simulink model "VehicleFollowing"  (R2020b)
settings: Solver=FixedStepAuto  StartTime=0.0  StopTime=23  FixedStep=Ts/2  RelTol=1e-3
PreLoadFcn:
  | VehicleFollowingInit;
values from neighbouring files (symbols this model uses):
  a_max = 2    [VehicleFollowingInit.m]
  a_min = -3    [VehicleFollowingInit.m]
  dimensionsEgo = [4; 2]    [VehicleFollowingInit.m]
  dimensionsLead = [6; 2]    [VehicleFollowingInit.m]
  dLead = 0    [VehicleFollowingInit.m]
  laneWidth = 3.7    [VehicleFollowingInit.m]
  lookAheadDistance = 6    [VehicleFollowingInit.m]
  roadTrajectory = [s_min  0        0 ... (first row only)    [VehicleFollowingInit.m]
  sLead_0 = 60    [VehicleFollowingInit.m]
  Ts = 0.01    [VehicleFollowingInit.m]    (also in prepare_simulation.m)
  v_max = 30    [VehicleFollowingInit.m]
  v_min = 0    [VehicleFollowingInit.m]
  vEgo_0 = 15    [VehicleFollowingInit.m]
  vLead_0 = 10    [VehicleFollowingInit.m]
  vLead_ref = vLead_0    (= 10)    [VehicleFollowingInit.m]
  wheelBaseEgo = 3    [VehicleFollowingInit.m]
  wheelBaseLead = 4    [VehicleFollowingInit.m]
  xEgo_0 = positionEgo_0(1)    [VehicleFollowingInit.m]
  xLead_0 = positionLead_0(1)    [VehicleFollowingInit.m]
  yEgo_0 = positionEgo_0(2)    [VehicleFollowingInit.m]
  yLead_0 = positionLead_0(2)    [VehicleFollowingInit.m]
undefined symbols (not defined in the file or in its folder): yawEgo_0, yawLead_0
libraries: pid_lib x2, sim3dautolib x2, vrlib x2, simulink x2, robotmobilelib x1, robotalgslib x1, drivingvehiclecontroller x1, sim3dlib x1, mpcadaslib x1
settings Model: Creator=Mustafa  LastModifiedBy=manuel
settings SFSimCC: CustomCodeUndefinedFunction=UseInterfaceOnly

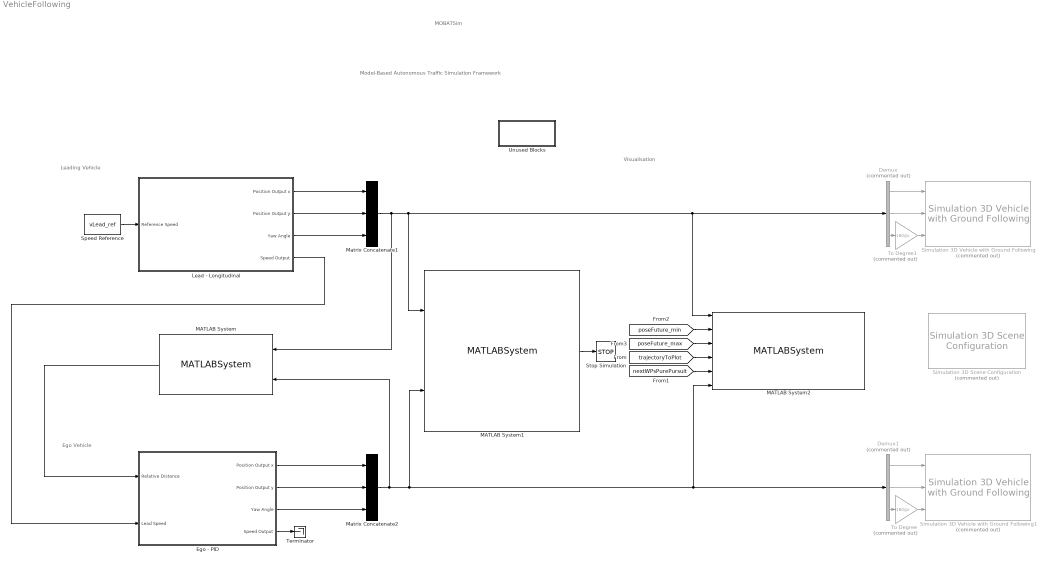
== system VehicleFollowing ==
  note: Visualisation
  note: Leading Vehicle
  note: Model-Based Autonomous Traffic Simulation Framework
  note: MOBATSim
  note: Ego Vehicle
  Demux : Demux  Commented=on  Outputs=3
  Demux1 : Demux  Commented=on  Outputs=3
  Ego - PID : Subsystem  mask{Speed=vEgo_0}
      mask prompts: Speed "Initial Speed"
      mask TypeOptions Speed: Initial Speed/Value
  Lead - Longitudinal : Subsystem  mask{s_0=sLead_0, d=dLead, Speed=vLead_0}
      mask prompts: s_0 "Initial s (Frenet)"; d "d (Frenet)"; Speed "Initial Speed"
      mask TypeOptions s_0: Initial Frenet s-coordinate/Value
      mask TypeOptions d: Frenet d-coordinate/Value
      mask TypeOptions Speed: Initial Speed/Value
  MATLAB System : MATLABSystem  System=RelativeFrenetDistance  LaneWidth=laneWidth  RoadTrajectory=roadTrajectory  SimulateUsing=Interpreted execution
      mask Type: RelativeFrenetDistance
      mask Display:
      | disp('RelativeFrenetDistance');
      | port_label('input',1,'poseLead');
      | port_label('input',2,'poseEgo');
      | port_label('output',1,'deltaS');
  MATLAB System1 : MATLABSystem  System=CollisionDetection  dimensionsEgo=dimensionsEgo  wheelBaseEgo=wheelBaseEgo  radiusEgo=radiusEgo  dimensionsLead=dimensionsLead  wheelBaseLead=wheelBaseLead  radiusLead=radiusLead  SimulateUsing=Interpreted execution
      mask Type: CollisionDetection
      mask Display:
      | disp('CollisionDetection');
      | port_label('input',1,'poseLead');
      | port_label('input',2,'poseEgo');
      | port_label('output',1,'collisionDetected');
  MATLAB System2 : MATLABSystem  System=PlotDrivingScenario  dimensionsLead=dimensionsLead  wheelBaseLead=wheelBaseLead  dimensionsEgo=dimensionsEgo  wheelBaseEgo=wheelBaseEgo  LaneWidth=laneWidth  RoadTrajectory=roadTrajectory  spaceDiscretisationMatrix=spaceDiscretisationMatrix  SimulateUsing=Interpreted execution
      mask Type: PlotDrivingScenario
      mask Display:
      | disp('PlotDrivingScenario');
      | port_label('input',1,'poseLead');
      | port_label('input',2,'poseLeadFuture_min');
      | port_label('input',3,'poseLeadFuture_max');
      | port_label('input',4,'egoTrajectory');
      | port_label('input',5,'nextWPsPurePursuit');
      | port_label('input',6,'poseEgo');
  Matrix Concatenate1 : Concatenate  NumInputs=3  ConcatenateDimension=2
  Matrix Concatenate2 : Concatenate  NumInputs=3  ConcatenateDimension=2
  Simulation 3D Scene Configuration : sim3dlib/Simulation 3D Scene Configuration  Priority=0  Commented=on  ProjectFormat=Default Scenes  SceneDesc=Straight road  ProjectName=VehicleSimulation.exe  ScenePath=/Game/Maps/HwStrght  vehTagList={'Scene Origin';'SimulinkVehicle1';'SimulinkVehicle2'}  vehTag=SimulinkVehicle2  OpVisEn=off  Ts=0.1  EnableWindow=on  sensorTag=MainCamera1  sensorId=1  sensorName=MainCamera1  mountLoc=Origin  offsetFlag=off  tmountOffset=[0, 0, 0]  rmountOffset=[0, 0, 0]  HorizontalResolution=1280  VerticalResolution=720  HorizontalFOV=60  mountPoint=[0 0 0]  mountOrientation=[0 0 0]  aMode=3  ID=1
      settings: SourceProductBaseCode=DR,UV,VE
  Simulation 3D Vehicle with Ground Following : sim3dautolib/Simulation 3D Vehicle with Ground Following  Priority=-1  Commented=on  PassVehMesh=Small pickup truck  VehColor=Orange  InitialPos=[xLead_0, yLead_0, yawLead_0]  InitialRot=[0, 0, 0]  ActorName=SimulinkVehicle1  SampleTime=0.1  ActorType=SimulinkVehicle  ID=1  aMode=3  ActorTag=SimulinkVehicle1  CoordinateScheme=ISO  TransformOutportEnabled=off
      settings: SourceProductBaseCode=DR,UV,VE
  Simulation 3D Vehicle with Ground Following1 : sim3dautolib/Simulation 3D Vehicle with Ground Following  Priority=-1  Commented=on  PassVehMesh=Muscle car  VehColor=Red  InitialPos=[xEgo_0, yEgo_0, yawEgo_0]  InitialRot=[0, 0, 0]  ActorName=SimulinkVehicle2  SampleTime=0.1  ActorType=SimulinkVehicle  ID=2  aMode=3  ActorTag=SimulinkVehicle2  CoordinateScheme=ISO  TransformOutportEnabled=off
      settings: SourceProductBaseCode=DR,UV,VE
  Speed Reference : Constant  Value=vLead_ref
  Stop Simulation : Stop
  Terminator : Terminator
  To Degree : Gain  Commented=on  Gain=180/pi
  To Degree1 : Gain  Commented=on  Gain=180/pi
  Unused Blocks : Subsystem
  wires:
  Speed Reference/1 -> Lead - Longitudinal/1(Reference Speed)
  Ego - PID/1(Position Output x) -> Matrix Concatenate2/1
  MATLAB System/1 -> Ego - PID/1(Relative Distance)
  Ego - PID/4(Speed Output) -> Terminator/1
  Ego - PID/2(Position Output y) -> Matrix Concatenate2/2
  Ego - PID/3(Yaw Angle) -> Matrix Concatenate2/3
  Matrix Concatenate1/1 -> Demux/1, MATLAB System2/1, MATLAB System1/1, MATLAB System/1
  Demux/1 -> Simulation 3D Vehicle with Ground Following/1
  Demux/2 -> Simulation 3D Vehicle with Ground Following/2
  Matrix Concatenate2/1 -> MATLAB System1/2, MATLAB System2/6, Demux1/1, MATLAB System/2
  Demux1/1 -> Simulation 3D Vehicle with Ground Following1/1
  Demux1/2 -> Simulation 3D Vehicle with Ground Following1/2
  Demux1/3 -> To Degree/1
  To Degree/1 -> Simulation 3D Vehicle with Ground Following1/3
  MATLAB System1/1 -> Stop Simulation/1
  Demux/3 -> To Degree1/1
  To Degree1/1 -> Simulation 3D Vehicle with Ground Following/3
  Lead - Longitudinal/1(Position Output x) -> Matrix Concatenate1/1
  Lead - Longitudinal/4(Speed Output) -> Ego - PID/2(Lead Speed)
  Lead - Longitudinal/3(Yaw Angle) -> Matrix Concatenate1/3
  Lead - Longitudinal/2(Position Output y) -> Matrix Concatenate1/2
  [nextWPsPurePursuit] -> MATLAB System2/5
  [trajectoryToPlot] -> MATLAB System2/4
  [poseFuture_min] -> MATLAB System2/2
  [poseFuture_max] -> MATLAB System2/3

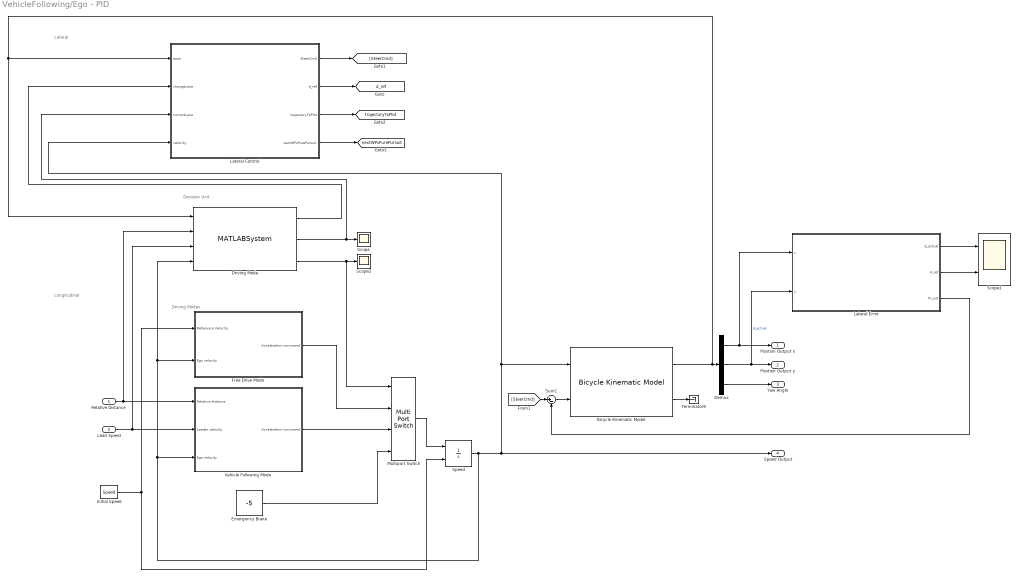
== system VehicleFollowing/Ego - PID ==
  note: Decision Unit
  note: Driving Modes
  note: Longitudinal
  note: Lateral
  Relative Distance : Inport
  Lead Speed : Inport  Port=2
  Bicycle Kinematic Model : robotmobilelib/Bicycle Kinematic Model  VehicleInputs=Vehicle Speed & Steering Angle  WheelBase=wheelBaseEgo  VehicleSpeedRange=[v_min v_max]  MaxSteeringAngle=steerAngle_max  InitialState=[xEgo_0; yEgo_0; yawEgo_0]  SimulateUsing=Interpreted execution
      settings: SourceProductBaseCode=RO
  Demux : Demux  Outputs=3
  Driving Mode : MATLABSystem  System=Decision  LaneWidth=laneWidth  RoadTrajectory=roadTrajectory  SimulateUsing=Interpreted execution
      mask Type: Decision
      mask Display:
      | disp('Decision');
      | port_label('input',1,'poseEgo');
      | port_label('input',2,'deltaS');
      | port_label('input',3,'vLead');
      | port_label('input',4,'vEgo');
      | port_label('output',1,'changeLaneCmd');
      | port_label('output',2,'currentLane');
      | port_label('output',3,'drivingMode');
  Emergency Brake : Constant  Value=-5
  Free Drive Mode : Subsystem
  Initial Speed : Constant  Value=Speed
  Lateral Control : Subsystem  Variant=on  VariantControlMode=label  LabelModeActiveChoice=STANLEY  mask{modeLateral=STANLEY}
      mask prompts: modeLateral "Lateral Mode:"
      mask TypeOptions modeLateral: PURE_PURSUIT | STANLEY
      mask Callback modeLateral: set_param(gcb,'OverrideUsingVariant',get_param(gcb,'modeLateral'))
  Lateral Error : Subsystem
  Multiport Switch : MultiPortSwitch
  Scope : Scope
  Scope1 : Scope  NumInputPorts=2
  Scope2 : Scope
  Speed : Integrator  InitialConditionSource=external  LimitOutput=on  UpperSaturationLimit=v_max  LowerSaturationLimit=v_min
  Sum1 : Sum  Inputs=|+-
  Terminator9 : Terminator
  Vehicle Following Mode : Subsystem
  Position Output x : Outport  VectorParamsAs1DForOutWhenUnconnected=off
  Position Output y : Outport  Port=2  VectorParamsAs1DForOutWhenUnconnected=off
  Yaw Angle : Outport  Port=3  VectorParamsAs1DForOutWhenUnconnected=off
  Speed Output : Outport  Port=4  VectorParamsAs1DForOutWhenUnconnected=off
  tag scope: d_ref=global, nextWPsPurePursuit=global, trajectoryToPlot=global
  wires:
  Initial Speed/1 -> Free Drive Mode/1(Reference Velocity), Speed/2
  Relative Distance/1 -> Driving Mode/2, Vehicle Following Mode/1(Relative distance)
  Lead Speed/1 -> Driving Mode/3, Vehicle Following Mode/2(Leader velocity)
  Vehicle Following Mode/1(Acceleration command) -> Multiport Switch/3
  Multiport Switch/1 -> Speed/1
  Free Drive Mode/1(Acceleration command) -> Multiport Switch/2
  Emergency Brake/1 -> Multiport Switch/4
  Driving Mode/3 -> Scope2/1, Multiport Switch/1
  Demux/3 -> Yaw Angle/1
  Bicycle Kinematic Model/2 -> Terminator9/1
  Demux/2 -> Position Output y/1, Lateral Error/2(y)  "d_actual"
  Driving Mode/2 -> Lateral Control/3(currentLane), Scope/1
  Lateral Control/1(SteerCmd) -> [SteerCmd]
  Lateral Control/2(d_ref) -> [d_ref]
  Driving Mode/1 -> Lateral Control/2(changeLane)
  Speed/1 -> Speed Output/1, Lateral Control/4(velocity), Bicycle Kinematic Model/1, Vehicle Following Mode/3(Ego velocity), Free Drive Mode/2(Ego velocity), Driving Mode/4
  Bicycle Kinematic Model/1 -> Driving Mode/1, Lateral Control/1(pose), Demux/1
  Lateral Control/3(trajectoryToPlot) -> [trajectoryToPlot]
  Lateral Control/4(nextWPsPurePursuit) -> [nextWPsPurePursuit]
  Sum1/1 -> Bicycle Kinematic Model/2
  [SteerCmd] -> Sum1/1
  Lateral Error/3(PI_out) -> Sum1/2
  Demux/1 -> Lateral Error/1(x), Position Output x/1
  Lateral Error/1(d_actual) -> Scope1/1
  Lateral Error/2(d_ref) -> Scope1/2

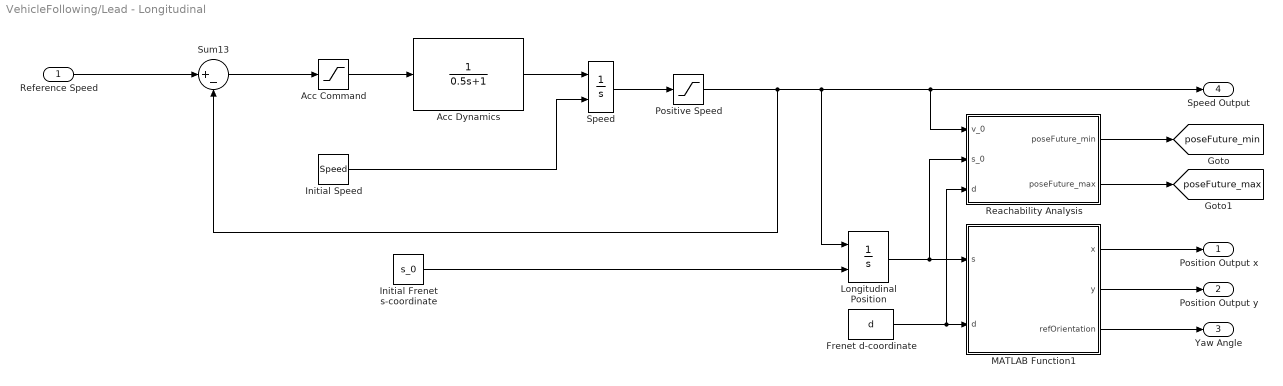
== system VehicleFollowing/Lead - Longitudinal ==
  Reference Speed : Inport
  Acc Command : Saturate  UpperLimit=a_max  LowerLimit=a_min
  Acc Dynamics : TransferFcn  Denominator=[0.5 1]
  Frenet d-coordinate : Constant  Value=d
  Initial Frenet s-coordinate : Constant  Value=s_0
  Initial Speed : Constant  Value=Speed
  Longitudinal Position : Integrator  InitialConditionSource=external
  MATLAB Function1 : MATLAB Function  TreatAsAtomicUnit=on  mask{currentTrajectory=roadTrajectory}
      mask prompts: currentTrajectory "Road trajectory"
  Positive Speed : Saturate  UpperLimit=v_max  LowerLimit=v_min
  Reachability Analysis : Subsystem
  Speed : Integrator  InitialConditionSource=external
  Sum13 : Sum  Inputs=|+-
  Position Output x : Outport  VectorParamsAs1DForOutWhenUnconnected=off
  Position Output y : Outport  Port=2
  Yaw Angle : Outport  Port=3
  Speed Output : Outport  Port=4  VectorParamsAs1DForOutWhenUnconnected=off
  tag scope: poseFuture_max=global, poseFuture_min=global
  wires:
  Speed/1 -> Positive Speed/1
  Positive Speed/1 -> Sum13/2, Reachability Analysis/1(v_0), Speed Output/1, Longitudinal Position/1
  Initial Frenet s-coordinate/1 -> Longitudinal Position/2
  Sum13/1 -> Acc Command/1
  Reference Speed/1 -> Sum13/1
  Acc Command/1 -> Acc Dynamics/1
  Acc Dynamics/1 -> Speed/1
  Initial Speed/1 -> Speed/2
  Frenet d-coordinate/1 -> Reachability Analysis/3(d), MATLAB Function1/2(d)
  Longitudinal Position/1 -> Reachability Analysis/2(s_0), MATLAB Function1/1(s)
  MATLAB Function1/1(x) -> Position Output x/1
  MATLAB Function1/2(y) -> Position Output y/1
  MATLAB Function1/3(refOrientation) -> Yaw Angle/1
  Reachability Analysis/1(poseFuture_min) -> [poseFuture_min]
  Reachability Analysis/2(poseFuture_max) -> [poseFuture_max]

== system VehicleFollowing/Unused Blocks ==
  note: V3
  note: Collision detecion
  3D Animation : Subsystem  Commented=on
  Collision Detection : Subsystem  Commented=on
  Driving Mode Selector : Stateflow chart  Commented=on  TreatAsAtomicUnit=on
  MATLAB Function : MATLAB Function  Commented=on  TreatAsAtomicUnit=on  SystemSampleTime=0.1  mask{dimensionsVehicle1=dimensionsLead, wheelBaseVehicle1=wheelBaseLead, dimensionsVehicle2=dimensionsEgo, wheelBaseVehicle2=wheelBaseEgo, LaneWidth=laneWidth, roadTrajectory=roadTrajectory}
      mask prompts: dimensionsVehicle1 "Dimensions (length, width) vehicle 1"; wheelBaseVehicle1 "Wheel base vehicle 1"; dimensionsVehicle2 "Dimensions (length, width) vehicle 2"; wheelBaseVehicle2 "Wheel base vehicle 2"; LaneWidth "Lane width"; roadTrajectory "Road trajectory according to MOBATSim map format"
      mask init:
      | close all;
      | figure('units','normalized','outerposition',[0 0 1 1]);
      | grid on
      | axis equal
      | hold on
  MPC : Subsystem  Commented=on  mask{Pos=20, Speed=25}
      mask prompts: Pos "Initial Position"; Speed "Initial Speed"
      mask TypeOptions Pos: Initial Position Z/Value
      mask TypeOptions Speed: Initial Speed/Value
  Steering Angle Ref : Constant  Commented=on  Value=0
  wires:
  Steering Angle Ref/1 -> MPC/3(Steering Angle Command)

== system VehicleFollowing/Ego - PID/Free Drive Mode ==
  Reference Velocity : Inport
  Ego velocity : Inport  Port=2
  Acc Command : Saturate  UpperLimit=v_max  LowerLimit=v_min
  Acc Dynamics : TransferFcn  Denominator=[0.5 1]
  Sum13 : Sum  Inputs=|+-
  Acceleration command : Outport
  wires:
  Sum13/1 -> Acc Command/1
  Acc Dynamics/1 -> Acceleration command/1
  Reference Velocity/1 -> Sum13/1
  Acc Command/1 -> Acc Dynamics/1
  Ego velocity/1 -> Sum13/2

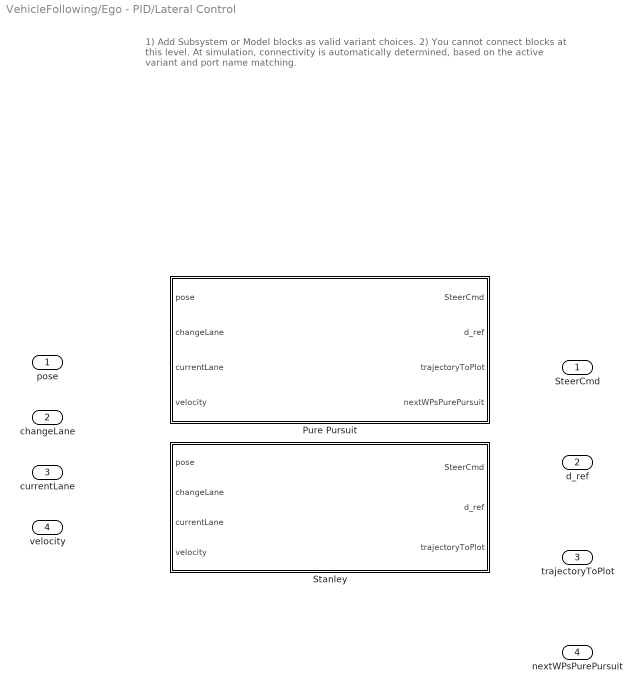
== system VehicleFollowing/Ego - PID/Lateral Control ==
  note: 1) Add Subsystem or Model blocks as valid variant choices.
      | 2) You cannot connect blocks at this level. At simulation, connectivity is automatically
      | determined, based on the active variant and port name matching.
  pose : Inport
  changeLane : Inport  Port=2
  currentLane : Inport  Port=3
  velocity : Inport  Port=4
  Pure Pursuit : Subsystem  VariantControl=PURE_PURSUIT
  Stanley : Subsystem  VariantControl=STANLEY
  SteerCmd : Outport
  d_ref : Outport  Port=2
  trajectoryToPlot : Outport  Port=3
  nextWPsPurePursuit : Outport  Port=4

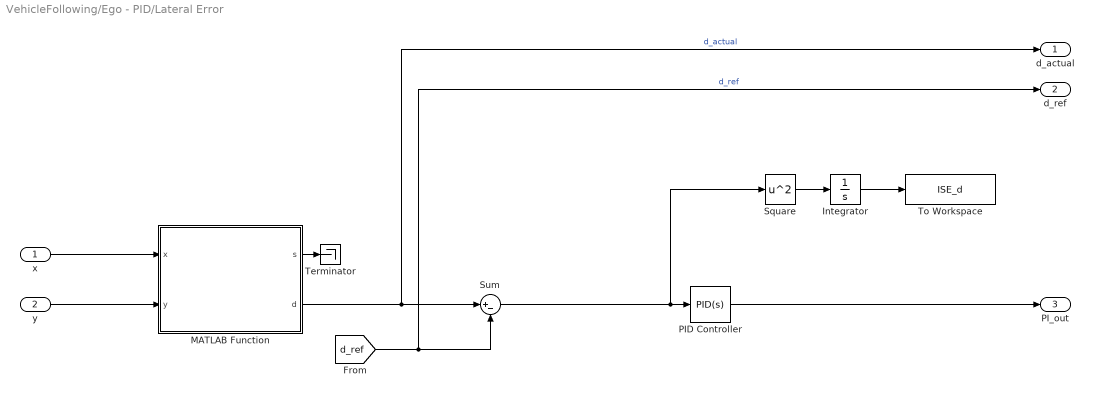
== system VehicleFollowing/Ego - PID/Lateral Error ==
  x : Inport
  y : Inport  Port=2
  Integrator : Integrator
  MATLAB Function : MATLAB Function  TreatAsAtomicUnit=on  mask{currentTrajectory=roadTrajectory}
      mask prompts: currentTrajectory "Road trajectory"
  PID Controller : pid_lib/PID Controller  Controller=PID  Form=Parallel  TimeDomain=Continuous-time  UseExternalTs=off  SampleTime=-1  IntegratorMethod=Forward Euler  FilterMethod=Forward Euler  ControllerParametersSource=internal  P=1  I=4  D=0  UseFilter=on  N=100  TunerSelectOption=Transfer Function Based (PID Tuner App)  InitialConditionSource=internal  InitialConditionForIntegrator=0  InitialConditionForFilter=0  DifferentiatorICPrevScaledInput=0  ExternalReset=none  TrackingMode=off  Kt=1  LimitOutput=off  SatLimitsSource=internal  UpperSaturationLimit=inf  LowerSaturationLimit=-inf  LinearizeAsGain=on  AntiWindupMode=none  Kb=1  POutMin=[]  POutMax=[]  IOutMin=[]  IOutMax=[]  DOutMin=[]  DOutMax=[]  NOutMin=[]  NOutMax=[]  SumOutMin=[]  SumOutMax=[]  SaturationOutMin=[]  SaturationOutMax=[]  PParamMin=[]  PParamMax=[]  IParamMin=[]  IParamMax=[]  DParamMin=[]  DParamMax=[]  NParamMin=[]  NParamMax=[]  KbParamMin=[]  KbParamMax=[]  KtParamMin=[]  KtParamMax=[]  KbOutMin=[]  KbOutMax=[]  KtOutMin=[]  KtOutMax=[]  IntegratorOutMin=[]  IntegratorOutMax=[]  FilterOutMin=[]  FilterOutMax=[]  SumI1OutMin=[]  SumI1OutMax=[]  SumI2OutMin=[]  SumI2OutMax=[]  SumI3OutMin=[]  SumI3OutMax=[]  SumI4OutMin=[]  SumI4OutMax=[]  SumDOutMin=[]  SumDOutMax=[]  DifferentiatorOutMin=[]  DifferentiatorOutMax=[]  FilterDiffOutCoefMin=[]  FilterDiffOutCoefMax=[]  ReciprocalOutMin=[]  ReciprocalOutMax=[]  SumDenOutMin=[]  SumDenOutMax=[]  SumNumOutMin=[]  SumNumOutMax=[]  DivideOutMin=[]  DivideOutMax=[]  UdiffTsProdOutMin=[]  UdiffTsProdOutMax=[]  NTsProdOutMin=[]  NTsProdOutMax=[]  UintegralTsProdOutMin=[]  UintegralTsProdOutMax=[]  UngainTsProdOutMin=[]  UngainTsProdOutMax=[]  IntegratorContinuousStateAttributes=''  IntegratorStateMustResolveToSignalObject=off  IntegratorRTWStateStorageClass=Auto  FilterContinuousStateAttributes=''  FilterStateMustResolveToSignalObject=off  FilterRTWStateStorageClass=Auto  ParallelPVariant=InternalParameters  IdealPVariant=Disabled  IVariant=InternalParameters  DVariant=InternalParameters  IntegratorVariant=Continuous  SatVariant=Disabled  AWVariant=Passthrough  PCopyVariant=Disabled  TRVariant=Disabled  FdbkBlocksVariant=Forward  IdealPFdbkVariant=Disabled  SatFdbkVariant=Disabled  DerivativeFilterVariant=ContFilter  NVariant=InternalParameters  NCopyVariant=Disabled  FilterICVariant=InternalICsFilter  IntegratorICVariant=InternalICs  ExternalResetVariant=Disabled  TRSumVariant=Passthrough  SumFdbkVariant=Disabled  SumVariant=Sum_PID  TsampFilterVariant=InternalTs  TsampNgainVariant=Passthrough  TsampIntegralVariant=Passthrough  ExternalSaturationOutDataTypeStr=Inherit: Same as second input
  Square : Math  Operator=square  SaturateOnIntegerOverflow=on
  Sum : Sum  Inputs=|+-
  Terminator : Terminator
  To Workspace : ToWorkspace  VariableName=ISE_d  SampleTime=-1
      settings: Save2DSignal=2-D array (concatenate along first dimension)
  d_actual : Outport
  d_ref : Outport  Port=2
  PI_out : Outport  Port=3
  wires:
  PID Controller/1 -> PI_out/1
  MATLAB Function/1(s) -> Terminator/1
  Integrator/1 -> To Workspace/1
  MATLAB Function/2(d) -> d_actual/1, Sum/1  "d_actual"
  [d_ref] -> d_ref/1, Sum/2  "d_ref"
  Sum/1 -> Square/1, PID Controller/1
  Square/1 -> Integrator/1
  y/1 -> MATLAB Function/2(y)
  x/1 -> MATLAB Function/1(x)

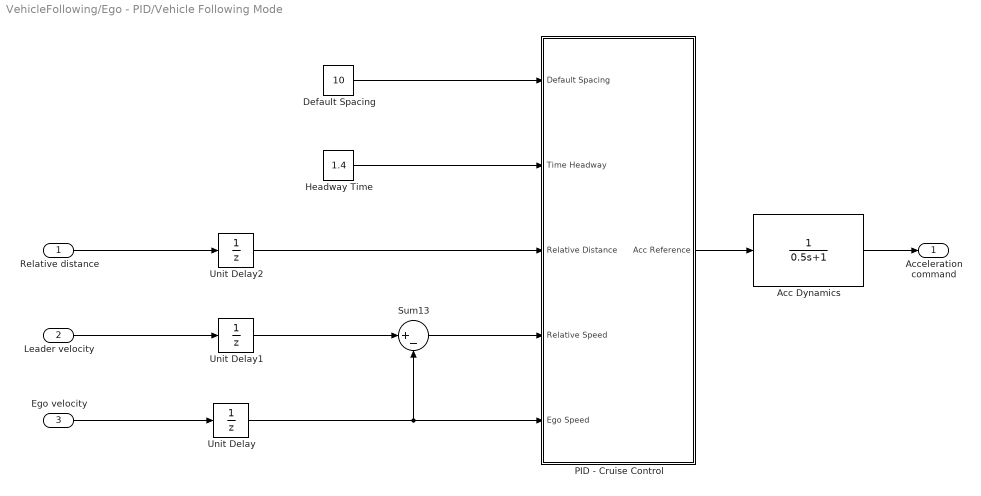
== system VehicleFollowing/Ego - PID/Vehicle Following Mode ==
  Relative distance : Inport
  Leader velocity : Inport  Port=2
  Ego velocity : Inport  Port=3
  Acc Dynamics : TransferFcn  Denominator=[0.5 1]
  Default Spacing : Constant  Value=10
  Headway Time : Constant  Value=1.4
  PID - Cruise Control : Subsystem
  Sum13 : Sum  Inputs=|+-
  Unit Delay : UnitDelay  SampleTime=-1  HasFrameUpgradeWarning=on
  Unit Delay1 : UnitDelay  SampleTime=-1  HasFrameUpgradeWarning=on
  Unit Delay2 : UnitDelay  SampleTime=-1  HasFrameUpgradeWarning=on
  Acceleration command : Outport
  wires:
  Leader velocity/1 -> Unit Delay1/1
  Headway Time/1 -> PID - Cruise Control/2(Time Headway)
  Ego velocity/1 -> Unit Delay/1
  Sum13/1 -> PID - Cruise Control/4(Relative Speed)
  Relative distance/1 -> Unit Delay2/1
  PID - Cruise Control/1(Acc Reference) -> Acc Dynamics/1
  Acc Dynamics/1 -> Acceleration command/1
  Default Spacing/1 -> PID - Cruise Control/1(Default Spacing)
  Unit Delay/1 -> Sum13/2, PID - Cruise Control/5(Ego Speed)
  Unit Delay1/1 -> Sum13/1
  Unit Delay2/1 -> PID - Cruise Control/3(Relative Distance)

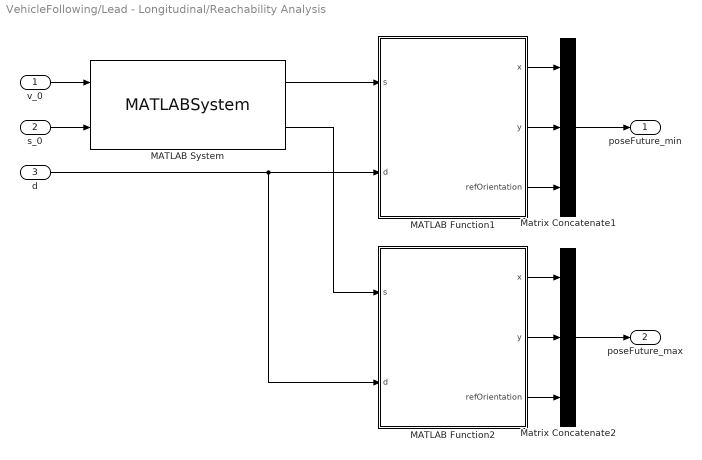
== system VehicleFollowing/Lead - Longitudinal/Reachability Analysis ==
  v_0 : Inport
  s_0 : Inport  Port=2
  d : Inport  Port=3
  MATLAB Function1 : MATLAB Function  TreatAsAtomicUnit=on  mask{currentTrajectory=roadTrajectory}
      mask prompts: currentTrajectory "Road trajectory"
  MATLAB Function2 : MATLAB Function  TreatAsAtomicUnit=on  mask{currentTrajectory=roadTrajectory}
      mask prompts: currentTrajectory "Road trajectory"
  MATLAB System : MATLABSystem  System=LongitudinalReachability  minimumAcceleration=a_min  maximumAcceleration=a_max  timeHorizon=timeHorizon  Ts=Ts  SimulateUsing=Interpreted execution
      mask Type: LongitudinalReachability
      mask Display:
      | disp('LongitudinalReachability');
      | port_label('input',1,'velocity_0');
      | port_label('input',2,'s_0');
      | port_label('output',1,'sFuture_min');
      | port_label('output',2,'sFuture_max');
  Matrix Concatenate1 : Concatenate  NumInputs=3  ConcatenateDimension=2
  Matrix Concatenate2 : Concatenate  NumInputs=3  ConcatenateDimension=2
  poseFuture_min : Outport
  poseFuture_max : Outport  Port=2
  wires:
  s_0/1 -> MATLAB System/2
  v_0/1 -> MATLAB System/1
  MATLAB System/1 -> MATLAB Function1/1(s)
  d/1 -> MATLAB Function2/2(d), MATLAB Function1/2(d)
  MATLAB System/2 -> MATLAB Function2/1(s)
  MATLAB Function1/1(x) -> Matrix Concatenate1/1
  MATLAB Function1/2(y) -> Matrix Concatenate1/2
  MATLAB Function1/3(refOrientation) -> Matrix Concatenate1/3
  MATLAB Function2/1(x) -> Matrix Concatenate2/1
  MATLAB Function2/2(y) -> Matrix Concatenate2/2
  MATLAB Function2/3(refOrientation) -> Matrix Concatenate2/3
  Matrix Concatenate1/1 -> poseFuture_min/1
  Matrix Concatenate2/1 -> poseFuture_max/1

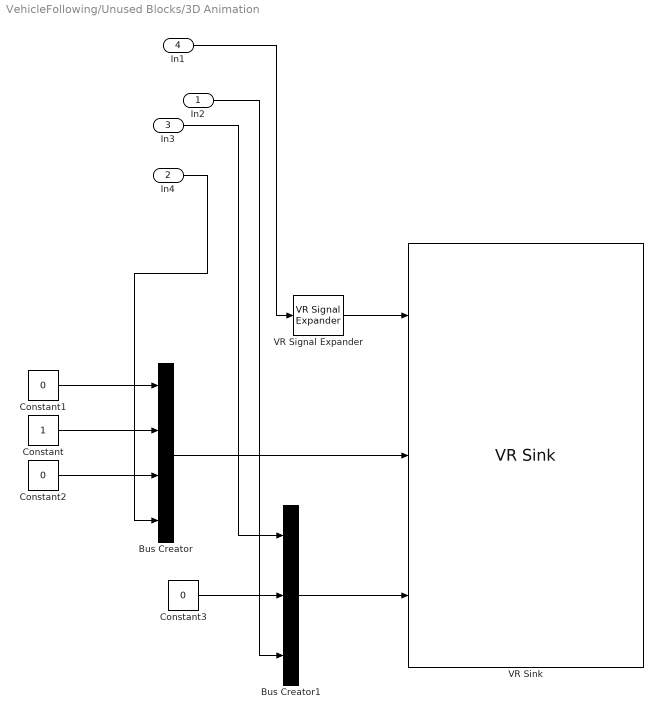
== system VehicleFollowing/Unused Blocks/3D Animation ==
  In2 : Inport
  In4 : Inport  Port=2
  In3 : Inport  Port=3
  In1 : Inport  Port=4
  Bus Creator : BusCreator  Inputs=4
  Bus Creator1 : BusCreator  Inputs=3
  Constant : Constant
  Constant1 : Constant  Value=0
  Constant2 : Constant  Value=0
  Constant3 : Constant  Value=0
  VR Signal Expander : vrlib/VR Signal Expander  outwidth=3  outidx=[3]
  VR Sink : vrlib/VR Sink  InstantiateOnLoad=on  SampleTime=0.02  ViewEnable=on  RemoteChange=off  RemoteView=off  FieldsWritten=Car_Red.translation.3.1.1.double#Car_Blue.rotation.4.1.1.double#Car_Blue.translation.3.1.1.double  WorldFileName=PlatoonWorld.WRL  AutoView=off  VideoDimensions=[]  AllowVariableSize=off
  wires:
  Constant/1 -> Bus Creator/2
  Constant1/1 -> Bus Creator/1
  Bus Creator1/1 -> VR Sink/3
  In2/1 -> Bus Creator1/3
  Bus Creator/1 -> VR Sink/2
  In4/1 -> Bus Creator/4
  In1/1 -> VR Signal Expander/1
  Constant3/1 -> Bus Creator1/2
  Constant2/1 -> Bus Creator/3
  VR Signal Expander/1 -> VR Sink/1
  In3/1 -> Bus Creator1/1

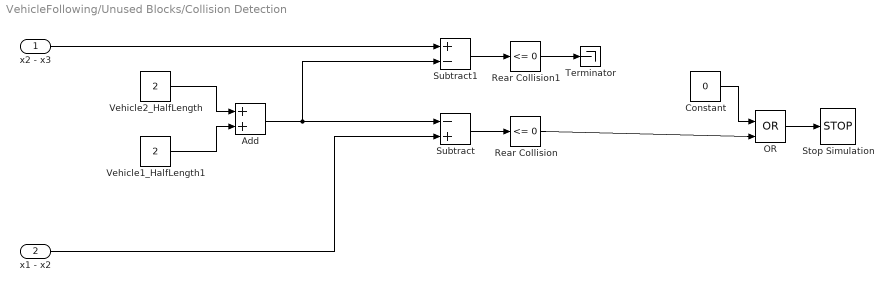
== system VehicleFollowing/Unused Blocks/Collision Detection ==
  x2 - x3 : Inport
  x1 - x2 : Inport  Port=2
  Add : Sum
  Constant : Constant  Value=0
  OR : Logic  Operator=OR  IconShape=distinctive  AllPortsSameDT=off  OutDataTypeStr=boolean
  Rear Collision : simulink/Logic and Bit Operations/Compare To Constant  relop=<=  const=0  OutDataTypeStr=boolean
  Rear Collision1 : simulink/Logic and Bit Operations/Compare To Constant  relop=<=  const=0  OutDataTypeStr=boolean
  Stop Simulation : Stop
  Subtract : Sum  Inputs=-+
  Subtract1 : Sum  Inputs=+-
  Terminator : Terminator
  Vehicle1_HalfLength1 : Constant  Value=2
  Vehicle2_HalfLength : Constant  Value=2
  wires:
  Vehicle2_HalfLength/1 -> Add/1
  OR/1 -> Stop Simulation/1
  Constant/1 -> OR/1
  Subtract1/1 -> Rear Collision1/1
  Add/1 -> Subtract1/2, Subtract/1
  Rear Collision1/1 -> Terminator/1
  Vehicle1_HalfLength1/1 -> Add/2
  Rear Collision/1 -> OR/2
  Subtract/1 -> Rear Collision/1
  x1 - x2/1 -> Subtract/2
  x2 - x3/1 -> Subtract1/1

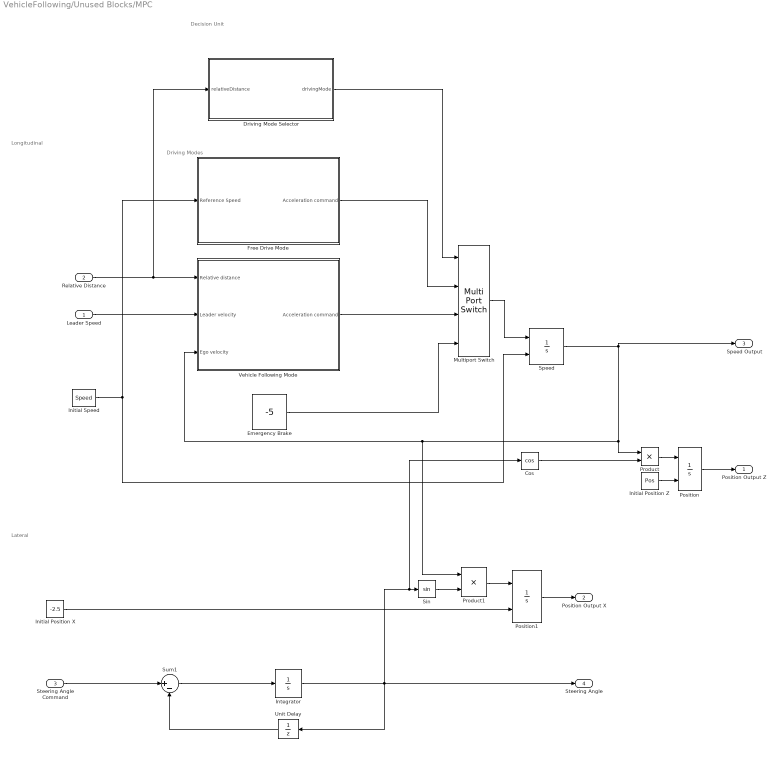
== system VehicleFollowing/Unused Blocks/MPC ==
  note: Decision Unit
  note: Driving Modes
  note: Longitudinal
  note: Lateral
  Leader Speed : Inport
  Relative Distance : Inport  Port=2
  Steering Angle Command : Inport  Port=3
  Cos : Trigonometry  Operator=cos
  Driving Mode Selector : Stateflow chart  TreatAsAtomicUnit=on
  Emergency Brake : Constant  Value=-5
  Free Drive Mode : Subsystem
  Initial Position X : Constant  Value=-2.5
  Initial Position Z : Constant  Value=Pos
  Initial Speed : Constant  Value=Speed
  Integrator : Integrator
  Multiport Switch : MultiPortSwitch
  Position : Integrator  InitialConditionSource=external
  Position1 : Integrator  InitialConditionSource=external
  Product : Product
  Product1 : Product
  Sin : Trigonometry
  Speed : Integrator  InitialConditionSource=external  LimitOutput=on  LowerSaturationLimit=0
  Sum1 : Sum  Inputs=|+-
  Unit Delay : UnitDelay  SampleTime=-1  HasFrameUpgradeWarning=on
  Vehicle Following Mode : Subsystem
  Position Output Z : Outport  VectorParamsAs1DForOutWhenUnconnected=off
  Position Output X : Outport  Port=2  VectorParamsAs1DForOutWhenUnconnected=off
  Speed Output : Outport  Port=3  VectorParamsAs1DForOutWhenUnconnected=off
  Steering Angle : Outport  Port=4  VectorParamsAs1DForOutWhenUnconnected=off
  wires:
  Position/1 -> Position Output Z/1
  Initial Speed/1 -> Free Drive Mode/1(Reference Speed), Speed/2
  Initial Position Z/1 -> Position/2
  Speed/1 -> Speed Output/1, Vehicle Following Mode/3(Ego velocity), Product1/1, Product/1
  Steering Angle Command/1 -> Sum1/1
  Sum1/1 -> Integrator/1
  Integrator/1 -> Unit Delay/1, Sin/1, Cos/1, Steering Angle/1
  Unit Delay/1 -> Sum1/2
  Initial Position X/1 -> Position1/2
  Cos/1 -> Product/2
  Product/1 -> Position/1
  Sin/1 -> Product1/2
  Product1/1 -> Position1/1
  Position1/1 -> Position Output X/1
  Relative Distance/1 -> Driving Mode Selector/1(relativeDistance), Vehicle Following Mode/1(Relative distance)
  Leader Speed/1 -> Vehicle Following Mode/2(Leader velocity)
  Vehicle Following Mode/1(Acceleration command) -> Multiport Switch/3
  Multiport Switch/1 -> Speed/1
  Free Drive Mode/1(Acceleration command) -> Multiport Switch/2
  Emergency Brake/1 -> Multiport Switch/4
  Driving Mode Selector/1(drivingMode) -> Multiport Switch/1

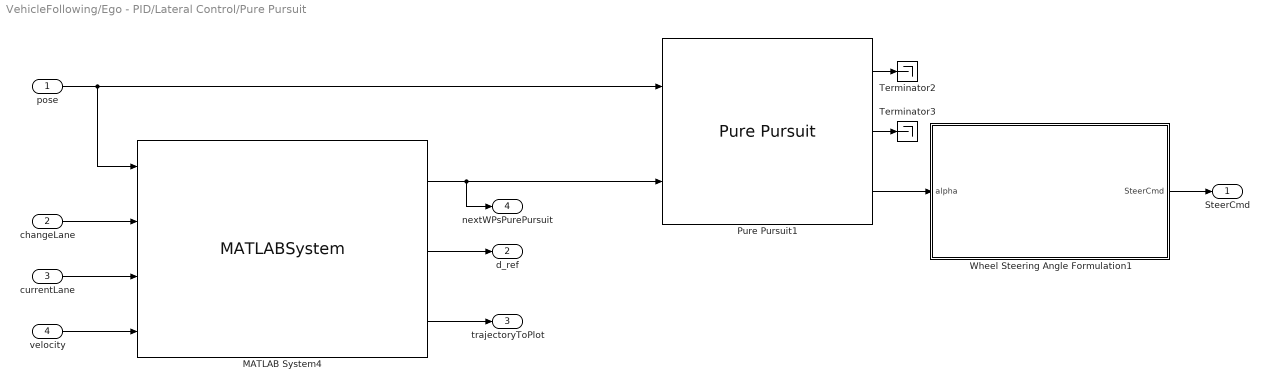
== system VehicleFollowing/Ego - PID/Lateral Control/Pure Pursuit ==
  pose : Inport
  changeLane : Inport  Port=2
  currentLane : Inport  Port=3
  velocity : Inport  Port=4
  MATLAB System4 : MATLABSystem  System=PurePursuitWPGenerator  numberWaypoints=numberWaypoints  LaneWidth=laneWidth  RoadTrajectory=roadTrajectory  durationToLeftLane=durationToLeftLane  durationToRightLane=durationToRightLane  timeHorizon=timeHorizon  Ts=Ts  SimulateUsing=Interpreted execution
      mask Type: PurePursuitWPGenerator
      mask Display:
      | disp('PurePursuitWPGenerator');
      | port_label('input',1,'pose');
      | port_label('input',2,'changeLaneCmd');
      | port_label('input',3,'currentLane');
      | port_label('input',4,'velocity');
      | port_label('output',1,'nextWPs');
      | port_label('output',2,'d_ref');
      | port_label('output',3,'trajectoryToPlot');
  Pure Pursuit1 : robotalgslib/Pure Pursuit  DesiredLinearVelocity=vEgo_0  MaxAngularVelocity=angularVelocity_max  LookaheadDistance=lookAheadDistance  TargetDirPort=on  SimulateUsing=Code generation
  Terminator2 : Terminator
  Terminator3 : Terminator
  Wheel Steering Angle Formulation1 : Subsystem
  SteerCmd : Outport
  d_ref : Outport  Port=2
  trajectoryToPlot : Outport  Port=3
  nextWPsPurePursuit : Outport  Port=4
  wires:
  Pure Pursuit1/1 -> Terminator2/1
  pose/1 -> Pure Pursuit1/1, MATLAB System4/1
  MATLAB System4/1 -> nextWPsPurePursuit/1, Pure Pursuit1/2
  Pure Pursuit1/3 -> Wheel Steering Angle Formulation1/1(alpha)
  Pure Pursuit1/2 -> Terminator3/1
  MATLAB System4/2 -> d_ref/1
  changeLane/1 -> MATLAB System4/2
  Wheel Steering Angle Formulation1/1(SteerCmd) -> SteerCmd/1
  velocity/1 -> MATLAB System4/4
  currentLane/1 -> MATLAB System4/3
  MATLAB System4/3 -> trajectoryToPlot/1

== system VehicleFollowing/Ego - PID/Lateral Control/Stanley ==
  pose : Inport
  changeLane : Inport  Port=2
  currentLane : Inport  Port=3
  velocity : Inport  Port=4
  Constant1 : Constant
  Lateral Controller Stanley1 : drivingvehiclecontroller/Lateral Controller Stanley  ModelType=Kinematic bicycle model  PositionGainF=2.5  PositionGainR=2.5  YawRateGain=0.2  DelayGain=0.2  VehicleMass=1575  Lf=1.2  Lr=1.6  TireStiffness=19000  Wheelbase=wheelBaseEgo  MaxSteeringAngle=steerAngle_max
      settings: SourceProductBaseCode=DR
  MATLAB System3 : MATLABSystem  System=StanleyPoseGenerator  wheelBase=wheelBaseEgo  LaneWidth=laneWidth  RoadTrajectory=roadTrajectory  durationToLeftLane=durationToLeftLane  durationToRightLane=durationToRightLane  timeHorizon=timeHorizon  Ts=Ts  SimulateUsing=Interpreted execution
      mask Type: StanleyPoseGenerator
      mask Display:
      | disp('StanleyPoseGenerator');
      | port_label('input',1,'pose');
      | port_label('input',2,'changeLaneCmd');
      | port_label('input',3,'currentLane');
      | port_label('input',4,'velocity');
      | port_label('output',1,'d_ref');
      | port_label('output',2,'trajectoryToPlot');
      | port_label('output',3,'referencePose');
      | port_label('output',4,'poseOut');
  SteerCmd : Outport
  d_ref : Outport  Port=2
  trajectoryToPlot : Outport  Port=3
  wires:
  MATLAB System3/4 -> Lateral Controller Stanley1/2
  Lateral Controller Stanley1/1 -> SteerCmd/1
  changeLane/1 -> MATLAB System3/2
  pose/1 -> MATLAB System3/1
  MATLAB System3/1 -> d_ref/1
  Constant1/1 -> Lateral Controller Stanley1/4
  velocity/1 -> Lateral Controller Stanley1/3, MATLAB System3/4
  currentLane/1 -> MATLAB System3/3
  MATLAB System3/3 -> Lateral Controller Stanley1/1
  MATLAB System3/2 -> trajectoryToPlot/1

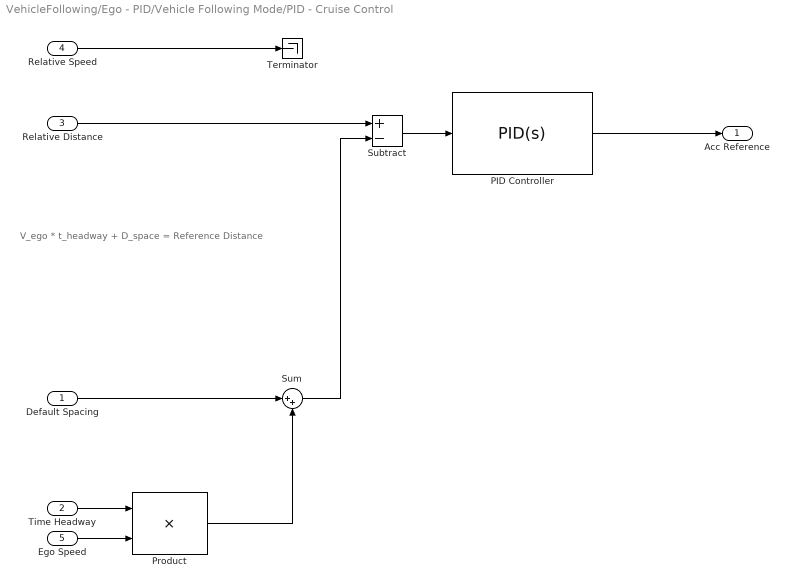
== system VehicleFollowing/Ego - PID/Vehicle Following Mode/PID - Cruise Control ==
  note: V_ego * t_headway + D_space = Reference Distance
  Default Spacing : Inport
  Time Headway : Inport  Port=2
  Relative Distance : Inport  Port=3
  Relative Speed : Inport  Port=4
  Ego Speed : Inport  Port=5
  PID Controller : pid_lib/PID Controller  Controller=PID  Form=Parallel  TimeDomain=Continuous-time  UseExternalTs=off  SampleTime=-1  IntegratorMethod=Forward Euler  FilterMethod=Forward Euler  ControllerParametersSource=internal  P=2  I=0.04  D=2.1  UseFilter=on  N=230  TunerSelectOption=Transfer Function Based (PID Tuner App)  InitialConditionSource=internal  InitialConditionForIntegrator=0  InitialConditionForFilter=0  DifferentiatorICPrevScaledInput=0  ExternalReset=none  TrackingMode=off  Kt=1  LimitOutput=on  SatLimitsSource=internal  UpperSaturationLimit=2  LowerSaturationLimit=-3  LinearizeAsGain=on  AntiWindupMode=clamping  Kb=1  POutMin=[]  POutMax=[]  IOutMin=[]  IOutMax=[]  DOutMin=[]  DOutMax=[]  NOutMin=[]  NOutMax=[]  SumOutMin=[]  SumOutMax=[]  SaturationOutMin=[]  SaturationOutMax=[]  PParamMin=[]  PParamMax=[]  IParamMin=[]  IParamMax=[]  DParamMin=[]  DParamMax=[]  NParamMin=[]  NParamMax=[]  KbParamMin=[]  KbParamMax=[]  KtParamMin=[]  KtParamMax=[]  KbOutMin=[]  KbOutMax=[]  KtOutMin=[]  KtOutMax=[]  IntegratorOutMin=[]  IntegratorOutMax=[]  FilterOutMin=[]  FilterOutMax=[]  SumI1OutMin=[]  SumI1OutMax=[]  SumI2OutMin=[]  SumI2OutMax=[]  SumI3OutMin=[]  SumI3OutMax=[]  SumI4OutMin=[]  SumI4OutMax=[]  SumDOutMin=[]  SumDOutMax=[]  DifferentiatorOutMin=[]  DifferentiatorOutMax=[]  FilterDiffOutCoefMin=[]  FilterDiffOutCoefMax=[]  ReciprocalOutMin=[]  ReciprocalOutMax=[]  SumDenOutMin=[]  SumDenOutMax=[]  SumNumOutMin=[]  SumNumOutMax=[]  DivideOutMin=[]  DivideOutMax=[]  UdiffTsProdOutMin=[]  UdiffTsProdOutMax=[]  NTsProdOutMin=[]  NTsProdOutMax=[]  UintegralTsProdOutMin=[]  UintegralTsProdOutMax=[]  UngainTsProdOutMin=[]  UngainTsProdOutMax=[]  IntegratorContinuousStateAttributes=''  IntegratorStateMustResolveToSignalObject=off  IntegratorRTWStateStorageClass=Auto  FilterContinuousStateAttributes=''  FilterStateMustResolveToSignalObject=off  FilterRTWStateStorageClass=Auto  ParallelPVariant=InternalParameters  IdealPVariant=Disabled  IVariant=InternalParameters  DVariant=InternalParameters  IntegratorVariant=Continuous  SatVariant=Enabled  AWVariant=ContClampingParallel  PCopyVariant=Disabled  TRVariant=Disabled  FdbkBlocksVariant=Forward  IdealPFdbkVariant=Disabled  SatFdbkVariant=Disabled  DerivativeFilterVariant=ContFilter  NVariant=InternalParameters  NCopyVariant=Disabled  FilterICVariant=InternalICsFilter  IntegratorICVariant=InternalICs  ExternalResetVariant=Disabled  TRSumVariant=Passthrough  SumFdbkVariant=Disabled  SumVariant=Sum_PID  TsampFilterVariant=InternalTs  TsampNgainVariant=Passthrough  TsampIntegralVariant=Passthrough  ExternalSaturationOutDataTypeStr=Inherit: Same as second input
  Product : Product
  Subtract : Sum  Inputs=+-
  Sum : Sum  Inputs=|++
  Terminator : Terminator
  Acc Reference : Outport
  wires:
  Ego Speed/1 -> Product/2
  Time Headway/1 -> Product/1
  Default Spacing/1 -> Sum/1
  Product/1 -> Sum/2
  Sum/1 -> Subtract/2
  Relative Distance/1 -> Subtract/1
  Subtract/1 -> PID Controller/1
  PID Controller/1 -> Acc Reference/1
  Relative Speed/1 -> Terminator/1

== system VehicleFollowing/Unused Blocks/MPC/Free Drive Mode ==
  Reference Speed : Inport
  Acc Command : Saturate  UpperLimit=2  LowerLimit=-3
  Acc Dynamics : TransferFcn  Denominator=[0.5 1]
  Sum13 : Sum  Inputs=|+-
  Acceleration command : Outport
  wires:
  Sum13/1 -> Acc Command/1
  Acc Dynamics/1 -> Acceleration command/1, Sum13/2
  Reference Speed/1 -> Sum13/1
  Acc Command/1 -> Acc Dynamics/1

== system VehicleFollowing/Unused Blocks/MPC/Vehicle Following Mode ==
  Relative distance : Inport
  Leader velocity : Inport  Port=2
  Ego velocity : Inport  Port=3
  Acc Dynamics : TransferFcn  Denominator=[0.5 1]
  Adaptive Cruise Control System : mpcadaslib/Adaptive Cruise Control System  EgoModel=tf(1,[0.5,1,0])  InitialEgoVelocity=30  DefaultSpacing=10  MaxVelocity=50  MinAcceleration=-3  amin_ext=off  MaxAcceleration=2  amax_ext=off  Ts=0.5  PredictionHorizon=200  ControllerBehavior=0.590  suboptimal=off  maxiter=100  datatypeopt=double  optmode=off  trackmode=off
  Headway Time : Constant  Value=1.4
  Reference Velocity : Constant  Value=30
  Sum13 : Sum  Inputs=|+-
  Acceleration command : Outport
  wires:
  Leader velocity/1 -> Sum13/1
  Headway Time/1 -> Adaptive Cruise Control System/2
  Reference Velocity/1 -> Adaptive Cruise Control System/1
  Ego velocity/1 -> Adaptive Cruise Control System/3, Sum13/2
  Sum13/1 -> Adaptive Cruise Control System/5
  Relative distance/1 -> Adaptive Cruise Control System/4
  Adaptive Cruise Control System/1 -> Acc Dynamics/1
  Acc Dynamics/1 -> Acceleration command/1

== system VehicleFollowing/Ego - PID/Lateral Control/Pure Pursuit/Wheel Steering Angle Formulation1 ==
  note: $\delta(t)=tan^{-1} \left( \frac{2\ L\ sin(\alpha)}{l_{d}} \right)$
  alpha : Inport
  Atan : Trigonometry  Operator=tan
  Divide : Product  Inputs=*/
  Gain : Gain  Gain=2
  One over Look Ahead Distance : Constant  Value=lookAheadDistance
  Product : Product
  Sine Wave : Sin  TimeSource=Use external signal  SampleTime=0
  Vehicle Length : Constant  Value=dimensionsEgo(1)
  SteerCmd : Outport
  wires:
  Vehicle Length/1 -> Gain/1
  Gain/1 -> Product/1
  alpha/1 -> Sine Wave/1
  Sine Wave/1 -> Product/2
  Product/1 -> Divide/1
  One over Look Ahead Distance/1 -> Divide/2
  Divide/1 -> Atan/1
  Atan/1 -> SteerCmd/1

== stateflow chart VehicleFollowing/Unused Blocks/Driving Mode Selector ==
  state VehicleFollowing
    entry:
    drivingMode = 2;
  state FreeDrive
    entry:
    drivingMode = 1;
  state EmergecyBrake
    entry:
    drivingMode = 3;
  (default) -> FreeDrive
  VehicleFollowing -> FreeDrive [order 1] : [relativeDistance > 50]
  FreeDrive -> VehicleFollowing [order 1] : [relativeDistance <= 40]
  FreeDrive -> EmergecyBrake [order 2] : [relativeDistance <= 10]
  VehicleFollowing -> EmergecyBrake [order 2] : [relativeDistance <= 10]
  EmergecyBrake -> VehicleFollowing : [relativeDistance > 15]
  data: relativeDistance input; drivingMode output

== matlab function VehicleFollowing/Lead - Longitudinal/MATLAB Function1 ==
  data: x output; y output; s input; d input; refOrientation output; currentTrajectory parameter
function [x, y, refOrientation] = Frenet2CartesianBlock(s, d, currentTrajectory)
% Simulink block for Frenet2Cartesian
    
    [position, refOrientation] = Frenet2Cartesian(s, d, currentTrajectory);
    x = position(1);
    y = position(2);
end

== stateflow chart VehicleFollowing/Unused Blocks/MPC/Driving Mode Selector ==
  state VehicleFollowing
    entry:
    drivingMode=2;
  state FreeDrive
    entry:
    drivingMode =1;
  state EmergecyBrake
    entry:
    drivingMode=3;
  (default) -> FreeDrive
  VehicleFollowing -> FreeDrive [order 1] : [relativeDistance >50]
  FreeDrive -> VehicleFollowing [order 1] : [relativeDistance <=40]
  FreeDrive -> EmergecyBrake [order 2] : [relativeDistance <=10]
  VehicleFollowing -> EmergecyBrake [order 2] : [relativeDistance <=10]
  EmergecyBrake -> VehicleFollowing : [relativeDistance>15]
  data: relativeDistance input; drivingMode output

== matlab function VehicleFollowing/Unused Blocks/MATLAB Function ==
  data: poseVehicle1 input; egoTrajectory input; nextWpsPurePursuit input; poseVehicle2 input; dimensionsVehicle1 parameter; wheelBaseVehicle1 parameter; dimensionsVehicle2 parameter; wheelBaseVehicle2 parameter; LaneWidth parameter; roadTrajectory parameter
function plotVehicles(poseVehicle1, egoTrajectory, nextWpsPurePursuit, poseVehicle2, dimensionsVehicle1, wheelBaseVehicle1, dimensionsVehicle2, wheelBaseVehicle2, LaneWidth, roadTrajectory)
% Plot vehicles and road and trajectory followed by the ego vehicle
    
    % Clear previous Vehicle
    cla;
    
    % Vehicle 1
    [plotVehicle1, plotVehicleLocation1] = plotVehicle(poseVehicle1, wheelBaseVehicle1, dimensionsVehicle1, 'g', 'o');
    % Traces
    
    
    % Vehicle 2
    [plotVehicle2, plotVehicleLocation2] = plotVehicle(poseVehicle2, wheelBaseVehicle2, dimensionsVehicle2, 'r', 'o');
    
    % Road 
    plotRoad(roadTrajectory, LaneWidth);
    
    % Trajectory
    plotTrajectory = plot(egoTrajectory(:, 1), egoTrajectory(:, 2), 'Color', 'green');
    plotWPs = plot(nextWpsPurePursuit(:, 1), nextWpsPurePursuit(:, 2), '-*');

    % Adjust Axis
    x2 = poseVehicle2(1);
    y2 = poseVehicle2(2);
    axis([x2-40 x2+40 y2-20 y2+20]); % Camera following V2 as ego vehicle
end

function [plotVehicle, plotVehicleLocation] = plotVehicle(poseRearAxle, wheelBase, dim, color, originRepresentation)
% Plot vehicle

    centerPoint = getVehicleCenterPoint(poseRearAxle, wheelBase);

    [corners_x, corners_y, ~] = createRectangleVehicle(centerPoint, poseRearAxle(3), dim);
    
    plotVehicle = plot(corners_x, corners_y, color); % Vehicle rectangle
    plotVehicleLocation = plot(poseRearAxle(1), poseRearAxle(2), originRepresentation, 'Color', 'black'); % Vehicle location
end

function plotRoad(roadTrajectory, laneWidth)
% Plot road

    route = roadTrajectory([1, 2],[1, 3]).*[1, -1; 1, -1];
    radian = roadTrajectory(3, 1);
    startPoint = route(1, :);
    endPoint = route(2, :);
    
    lineOffset = -laneWidth/2; % Offset for each line: Start with lower line

    if radian == 0 % Straight road
        route_Vector = endPoint - startPoint;
        routeUnitVector = route_Vector/norm(route_Vector);% unit vector of the route_vector
        routeNormalUnitVector = [-routeUnitVector(2), routeUnitVector(1)]; % Route normal unit vector

        for lineNr = 1:3 % For lower, middle and upper line
            startLine = startPoint + lineOffset*routeNormalUnitVector;
            endLine = endPoint + lineOffset*routeNormalUnitVector;
            
            lineOffset = plotRoadLine([startLine(1), endLine(1)], [startLine(2), endLine(2)], lineNr, lineOffset, laneWidth);
        end
    else % Curved road
        rotationCenter = roadTrajectory(3, [2, 3]).*[1, -1]; 
        startPointVector = startPoint - rotationCenter;
        routeRadius = norm(startPointVector); 
        startPointVectorAng = atan2(startPointVector(2),startPointVector(1)); 

        angles = startPointVectorAng:radian/(0.2*routeRadius*radian/pi):startPointVectorAng+radian; % Discretise angles from start to end point

        for lineNr = 1:3 % For lower, middle and upper line
            x_arc = rotationCenter(1) + (routeRadius-lineOffset)*cos(angles);
            y_arc = rotationCenter(2) + (routeRadius-lineOffset)*sin(angles);
            
            lineOffset = plotRoadLine(x_arc, y_arc, lineNr, lineOffset, laneWidth);
        end  
    end
end

function lineOffset = plotRoadLine(x_line, y_line, lineNr, lineOffset, laneWidth)
% Plot current road line, return offset for next line

    lineRepresentation = '-';
    if lineNr == 2 % Dashed for middle line
        lineRepresentation = '--';
    end

    plot(x_line, y_line, lineRepresentation, 'Color', 'blue');
    
    lineOffset = lineOffset + laneWidth; % Next line
end

== matlab function VehicleFollowing/Ego - PID/Lateral Error/MATLAB Function ==
  data: s output; x input; y input; d output; currentTrajectory parameter
function [s, d] = Cartesian2FrenetBlock(x, y, currentTrajectory)
% Simulink block for Frenet2Cartesian

    [s, d] = Cartesian2Frenet(currentTrajectory, [x, y]);
end

== matlab function VehicleFollowing/Lead - Longitudinal/Reachability Analysis/MATLAB Function1 ==
  data: x output; y output; s input; d input; refOrientation output; currentTrajectory parameter
function [x, y, refOrientation] = Frenet2CartesianBlock(s, d, currentTrajectory)
% Simulink block for Frenet2Cartesian
    
    [position, refOrientation] = Frenet2Cartesian(s, d, currentTrajectory);
    x = position(1);
    y = position(2);
end

== matlab function VehicleFollowing/Lead - Longitudinal/Reachability Analysis/MATLAB Function2 ==
  data: x output; y output; s input; d input; refOrientation output; currentTrajectory parameter
function [x, y, refOrientation] = Frenet2CartesianBlock(s, d, currentTrajectory)
% Simulink block for Frenet2Cartesian
    
    [position, refOrientation] = Frenet2Cartesian(s, d, currentTrajectory);
    x = position(1);
    y = position(2);
end
